simulink model "PhysicalEverSimmer"  (R2026a)
settings: Solver=VariableStepAuto  StopTime=14400
undefined symbols (not defined in the file): ES_PackRate_bph, ES_PrepRate_bph, ES_QCRate_bph, ES_Resupply_bph, Fault_T_Cell1, Fault_T_Cell2, Fault_T_Cell3, Recipe_Block_s, Recipe_Count, Resupply_Cutoff_T, Transport_Latency_s, Transport_Rate_bph
(part 2 of 2)

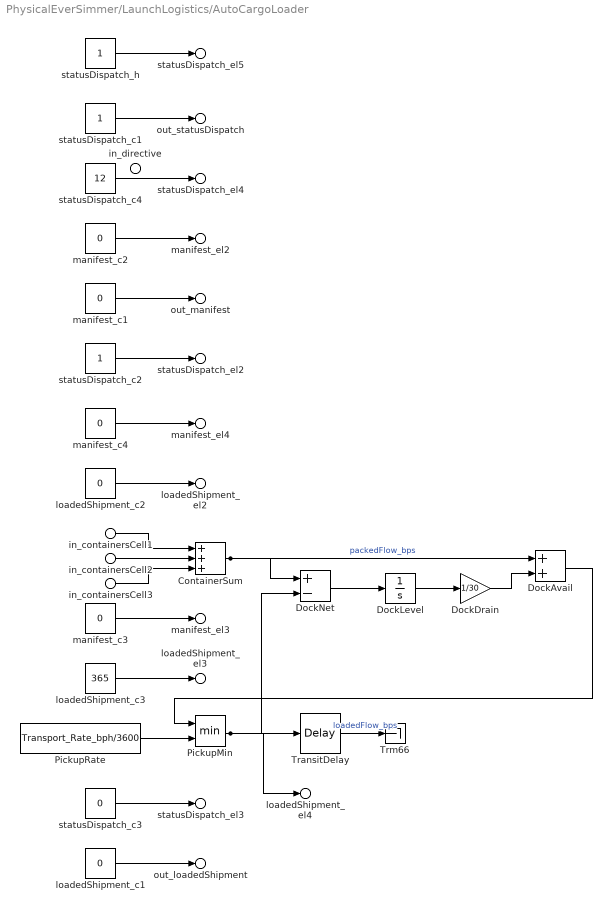
== system PhysicalEverSimmer/LaunchLogistics/AutoCargoLoader ==
  in_containersCell1 : Inport  PortName=containersCell1  Element=flow_bps
  in_containersCell2 : Inport  Port=2  PortName=containersCell2  Element=flow_bps
  in_containersCell3 : Inport  Port=3  PortName=containersCell3  Element=flow_bps
  in_directive : Inport  Port=4  PortName=directive
  ContainerSum : Sum  Inputs=+++
  DockAvail : Sum
  DockDrain : Gain  Gain=1/30
  DockLevel : Integrator  LimitOutput=on  UpperSaturationLimit=600  LowerSaturationLimit=0
  DockNet : Sum  Inputs=+-
  PickupMin : MinMax  Inputs=2
  PickupRate : Constant  Value=Transport_Rate_bph/3600
  TransitDelay : TransportDelay  DelayTime=Transport_Latency_s
  Trm66 : Terminator
  loadedShipment_c1 : Constant  Value=0
  loadedShipment_c2 : Constant  Value=0
  loadedShipment_c3 : Constant  Value=365
  manifest_c{1..4} (4 alike) : Constant  Value=0
  statusDispatch_c1 : Constant
  statusDispatch_c2 : Constant
  statusDispatch_c3 : Constant  Value=0
  statusDispatch_c4 : Constant  Value=12
  statusDispatch_h : Constant
  out_loadedShipment : Outport  PortName=loadedShipment  Element=batchId
  loadedShipment_el2 : Outport  PortName=loadedShipment  Element=count
  loadedShipment_el3 : Outport  PortName=loadedShipment  Element=sealRating_days
  loadedShipment_el4 : Outport  PortName=loadedShipment  Element=flow_bps
  out_manifest : Outport  Port=2  PortName=manifest  Element=destinationId
  manifest_el2 : Outport  Port=2  PortName=manifest  Element=batchId
  manifest_el3 : Outport  Port=2  PortName=manifest  Element=count
  manifest_el4 : Outport  Port=2  PortName=manifest  Element=mass_kg
  out_statusDispatch : Outport  Port=3  PortName=statusDispatch  Element=unitId
  statusDispatch_el2 : Outport  Port=3  PortName=statusDispatch  Element=opState
  statusDispatch_el3 : Outport  Port=3  PortName=statusDispatch  Element=faultCode
  statusDispatch_el4 : Outport  Port=3  PortName=statusDispatch  Element=power_kW
  statusDispatch_el5 : Outport  Port=3  PortName=statusDispatch  Element=health
  wires:
  manifest_c1/1 -> out_manifest/1
  statusDispatch_h/1 -> statusDispatch_el5/1
  statusDispatch_c1/1 -> out_statusDispatch/1
  statusDispatch_c4/1 -> statusDispatch_el4/1
  loadedShipment_c2/1 -> loadedShipment_el2/1
  manifest_c2/1 -> manifest_el2/1
  statusDispatch_c2/1 -> statusDispatch_el2/1
  manifest_c4/1 -> manifest_el4/1
  in_containersCell1/1 -> ContainerSum/1
  manifest_c3/1 -> manifest_el3/1
  in_containersCell2/1 -> ContainerSum/2
  in_containersCell3/1 -> ContainerSum/3
  loadedShipment_c3/1 -> loadedShipment_el3/1
  PickupRate/1 -> PickupMin/2
  loadedShipment_c1/1 -> out_loadedShipment/1
  statusDispatch_c3/1 -> statusDispatch_el3/1
  ContainerSum/1 -> DockAvail/1, DockNet/1  "packedFlow_bps"
  PickupMin/1 -> DockNet/2, TransitDelay/1, loadedShipment_el4/1
  DockNet/1 -> DockLevel/1
  TransitDelay/1 -> Trm66/1  "loadedFlow_bps"
  DockLevel/1 -> DockDrain/1
  DockDrain/1 -> DockAvail/2
  DockAvail/1 -> PickupMin/1

== system PhysicalEverSimmer/LaunchLogistics/AutoRefuelCell ==
  in_directive : Inport  PortName=directive
  statusRefuel_c1 : Constant
  statusRefuel_c2 : Constant
  statusRefuel_c3 : Constant  Value=0
  statusRefuel_c4 : Constant  Value=10
  statusRefuel_h : Constant
  out_statusRefuel : Outport  PortName=statusRefuel  Element=unitId
  statusRefuel_el2 : Outport  PortName=statusRefuel  Element=opState
  statusRefuel_el3 : Outport  PortName=statusRefuel  Element=faultCode
  statusRefuel_el4 : Outport  PortName=statusRefuel  Element=power_kW
  statusRefuel_el5 : Outport  PortName=statusRefuel  Element=health
  wires:
  statusRefuel_h/1 -> statusRefuel_el5/1
  statusRefuel_c3/1 -> statusRefuel_el3/1
  statusRefuel_c1/1 -> out_statusRefuel/1
  statusRefuel_c4/1 -> statusRefuel_el4/1
  statusRefuel_c2/1 -> statusRefuel_el2/1

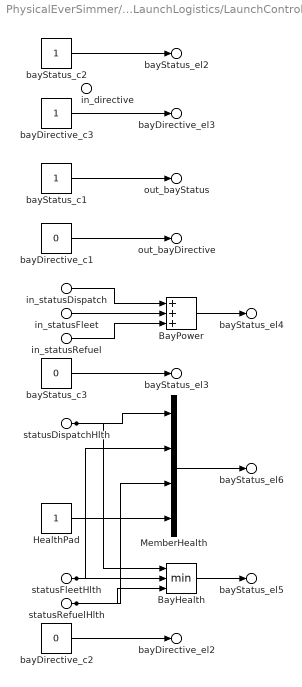
== system PhysicalEverSimmer/LaunchLogistics/LaunchController ==
  in_directive : Inport  PortName=directive
  in_statusDispatch : Inport  Port=2  PortName=statusDispatch  Element=power_kW
  statusDispatchHlth : Inport  Port=2  PortName=statusDispatch  Element=health
  in_statusRefuel : Inport  Port=3  PortName=statusRefuel  Element=power_kW
  statusRefuelHlth : Inport  Port=3  PortName=statusRefuel  Element=health
  in_statusFleet : Inport  Port=4  PortName=statusFleet  Element=power_kW
  statusFleetHlth : Inport  Port=4  PortName=statusFleet  Element=health
  BayHealth : MinMax  Inputs=3
  BayPower : Sum  Inputs=+++
  HealthPad : Constant
  MemberHealth : Mux
  bayDirective_c1 : Constant  Value=0
  bayDirective_c2 : Constant  Value=0
  bayDirective_c3 : Constant
  bayStatus_c1 : Constant
  bayStatus_c2 : Constant
  bayStatus_c3 : Constant  Value=0
  out_bayDirective : Outport  PortName=bayDirective  Element=cmdType
  bayDirective_el2 : Outport  PortName=bayDirective  Element=targetId
  bayDirective_el3 : Outport  PortName=bayDirective  Element=setpoint
  out_bayStatus : Outport  Port=2  PortName=bayStatus  Element=unitId
  bayStatus_el2 : Outport  Port=2  PortName=bayStatus  Element=opState
  bayStatus_el3 : Outport  Port=2  PortName=bayStatus  Element=faultCode
  bayStatus_el4 : Outport  Port=2  PortName=bayStatus  Element=power_kW
  bayStatus_el5 : Outport  Port=2  PortName=bayStatus  Element=health
  bayStatus_el6 : Outport  Port=2  PortName=bayStatus  Element=lineHealth
  wires:
  bayDirective_c1/1 -> out_bayDirective/1
  bayStatus_c2/1 -> bayStatus_el2/1
  bayDirective_c3/1 -> bayDirective_el3/1
  bayStatus_c1/1 -> out_bayStatus/1
  in_statusFleet/1 -> BayPower/2
  in_statusDispatch/1 -> BayPower/1
  bayStatus_c3/1 -> bayStatus_el3/1
  bayDirective_c2/1 -> bayDirective_el2/1
  in_statusRefuel/1 -> BayPower/3
  statusDispatchHlth/1 -> BayHealth/1, MemberHealth/1
  HealthPad/1 -> MemberHealth/4
  statusFleetHlth/1 -> BayHealth/2, MemberHealth/2
  statusRefuelHlth/1 -> BayHealth/3, MemberHealth/3
  BayPower/1 -> bayStatus_el4/1
  MemberHealth/1 -> bayStatus_el6/1
  BayHealth/1 -> bayStatus_el5/1

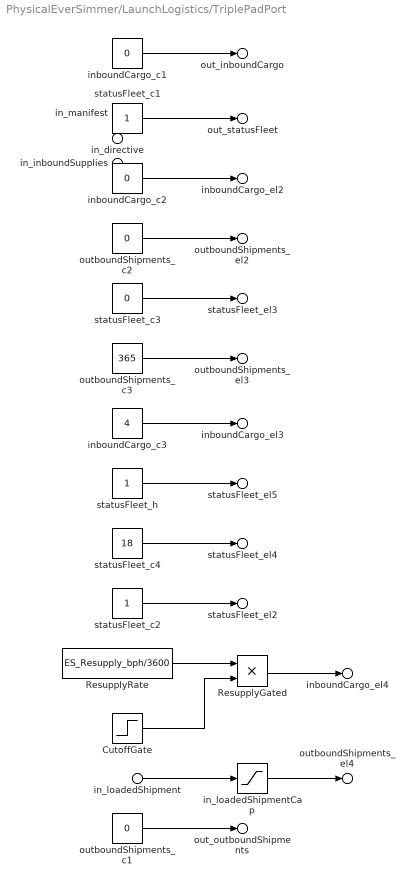
== system PhysicalEverSimmer/LaunchLogistics/TriplePadPort ==
  in_loadedShipment : Inport  PortName=loadedShipment  Element=flow_bps
  in_manifest : Inport  Port=2  PortName=manifest
  in_directive : Inport  Port=3  PortName=directive
  in_inboundSupplies : Inport  Port=4  PortName=inboundSupplies
  CutoffGate : Step  Time=Resupply_Cutoff_T  InitialValue=1  FinalValue=0  SampleTime=0
  ResupplyGated : Product
  ResupplyRate : Constant  Value=ES_Resupply_bph/3600
  in_loadedShipmentCap : Saturate  UpperLimit=0.0777777777778  LowerLimit=0
  inboundCargo_c1 : Constant  Value=0
  inboundCargo_c2 : Constant  Value=0
  inboundCargo_c3 : Constant  Value=4
  outboundShipments_c1 : Constant  Value=0
  outboundShipments_c2 : Constant  Value=0
  outboundShipments_c3 : Constant  Value=365
  statusFleet_c1 : Constant
  statusFleet_c2 : Constant
  statusFleet_c3 : Constant  Value=0
  statusFleet_c4 : Constant  Value=18
  statusFleet_h : Constant
  out_inboundCargo : Outport  PortName=inboundCargo  Element=palletId
  inboundCargo_el2 : Outport  PortName=inboundCargo  Element=mass_kg
  inboundCargo_el3 : Outport  PortName=inboundCargo  Element=temp_C
  inboundCargo_el4 : Outport  PortName=inboundCargo  Element=flow_bps
  out_outboundShipments : Outport  Port=2  PortName=outboundShipments  Element=batchId
  outboundShipments_el2 : Outport  Port=2  PortName=outboundShipments  Element=count
  outboundShipments_el3 : Outport  Port=2  PortName=outboundShipments  Element=sealRating_days
  outboundShipments_el4 : Outport  Port=2  PortName=outboundShipments  Element=flow_bps
  out_statusFleet : Outport  Port=3  PortName=statusFleet  Element=unitId
  statusFleet_el2 : Outport  Port=3  PortName=statusFleet  Element=opState
  statusFleet_el3 : Outport  Port=3  PortName=statusFleet  Element=faultCode
  statusFleet_el4 : Outport  Port=3  PortName=statusFleet  Element=power_kW
  statusFleet_el5 : Outport  Port=3  PortName=statusFleet  Element=health
  wires:
  inboundCargo_c1/1 -> out_inboundCargo/1
  statusFleet_c1/1 -> out_statusFleet/1
  statusFleet_h/1 -> statusFleet_el5/1
  inboundCargo_c2/1 -> inboundCargo_el2/1
  inboundCargo_c3/1 -> inboundCargo_el3/1
  outboundShipments_c2/1 -> outboundShipments_el2/1
  outboundShipments_c3/1 -> outboundShipments_el3/1
  statusFleet_c3/1 -> statusFleet_el3/1
  statusFleet_c4/1 -> statusFleet_el4/1
  statusFleet_c2/1 -> statusFleet_el2/1
  ResupplyRate/1 -> ResupplyGated/1
  CutoffGate/1 -> ResupplyGated/2
  in_loadedShipment/1 -> in_loadedShipmentCap/1
  outboundShipments_c1/1 -> out_outboundShipments/1
  ResupplyGated/1 -> inboundCargo_el4/1
  in_loadedShipmentCap/1 -> outboundShipments_el4/1

== system PhysicalEverSimmer/PlantServices/GravityCompMesh ==
  in_ambientGravity : Inport  PortName=ambientGravity  Element=gravity_g
  envStatus_c1 : Constant  Value=100
  out_envStatus : Outport  PortName=envStatus  Element=gravity_g
  envStatus_el2 : Outport  PortName=envStatus  Element=compensation_pct
  wires:
  in_ambientGravity/1 -> out_envStatus/1  "ambientGravity"
  envStatus_c1/1 -> envStatus_el2/1

== system PhysicalEverSimmer/PlantServices/RedundantReactorPair ==
  in_directive : Inport  PortName=directive
  statusPower_c1 : Constant
  statusPower_c2 : Constant
  statusPower_c3 : Constant  Value=0
  statusPower_c4 : Constant  Value=0
  statusPower_h : Constant
  out_statusPower : Outport  PortName=statusPower  Element=unitId
  statusPower_el2 : Outport  PortName=statusPower  Element=opState
  statusPower_el3 : Outport  PortName=statusPower  Element=faultCode
  statusPower_el4 : Outport  PortName=statusPower  Element=power_kW
  statusPower_el5 : Outport  PortName=statusPower  Element=health
  wires:
  statusPower_h/1 -> statusPower_el5/1
  statusPower_c3/1 -> statusPower_el3/1
  statusPower_c1/1 -> out_statusPower/1
  statusPower_c4/1 -> statusPower_el4/1
  statusPower_c2/1 -> statusPower_el2/1

== system PhysicalEverSimmer/PlantServices/RoboTransportSwarm ==
  in_transportDirective : Inport  PortName=transportDirective
  statusTransport_c1 : Constant
  statusTransport_c2 : Constant
  statusTransport_c3 : Constant  Value=0
  statusTransport_c4 : Constant  Value=15
  statusTransport_h : Constant
  out_statusTransport : Outport  PortName=statusTransport  Element=unitId
  statusTransport_el2 : Outport  PortName=statusTransport  Element=opState
  statusTransport_el3 : Outport  PortName=statusTransport  Element=faultCode
  statusTransport_el4 : Outport  PortName=statusTransport  Element=power_kW
  statusTransport_el5 : Outport  PortName=statusTransport  Element=health
  wires:
  statusTransport_h/1 -> statusTransport_el5/1
  statusTransport_c3/1 -> statusTransport_el3/1
  statusTransport_c1/1 -> out_statusTransport/1
  statusTransport_c4/1 -> statusTransport_el4/1
  statusTransport_c2/1 -> statusTransport_el2/1

== system PhysicalEverSimmer/PlantServices/ServicesController ==
  in_directive : Inport  PortName=directive
  in_statusPower : Inport  Port=2  PortName=statusPower  Element=power_kW
  statusPowerHlth : Inport  Port=2  PortName=statusPower  Element=health
  in_statusTransport : Inport  Port=3  PortName=statusTransport  Element=power_kW
  statusTransportHlth : Inport  Port=3  PortName=statusTransport  Element=health
  BayHealth : MinMax  Inputs=2
  BayPower : Sum
  HealthPad : Constant
  MemberHealth : Mux
  bayDirective_c1 : Constant  Value=0
  bayDirective_c2 : Constant  Value=0
  bayDirective_c3 : Constant
  bayStatus_c1 : Constant
  bayStatus_c2 : Constant
  bayStatus_c3 : Constant  Value=0
  out_bayDirective : Outport  PortName=bayDirective  Element=cmdType
  bayDirective_el2 : Outport  PortName=bayDirective  Element=targetId
  bayDirective_el3 : Outport  PortName=bayDirective  Element=setpoint
  out_bayStatus : Outport  Port=2  PortName=bayStatus  Element=unitId
  bayStatus_el2 : Outport  Port=2  PortName=bayStatus  Element=opState
  bayStatus_el3 : Outport  Port=2  PortName=bayStatus  Element=faultCode
  bayStatus_el4 : Outport  Port=2  PortName=bayStatus  Element=power_kW
  bayStatus_el5 : Outport  Port=2  PortName=bayStatus  Element=health
  bayStatus_el6 : Outport  Port=2  PortName=bayStatus  Element=lineHealth
  wires:
  bayStatus_c2/1 -> bayStatus_el2/1
  bayDirective_c3/1 -> bayDirective_el3/1
  statusPowerHlth/1 -> BayHealth/1, MemberHealth/1
  bayStatus_c1/1 -> out_bayStatus/1
  bayDirective_c1/1 -> out_bayDirective/1
  bayStatus_c3/1 -> bayStatus_el3/1
  in_statusPower/1 -> BayPower/1
  in_statusTransport/1 -> BayPower/2
  HealthPad/1 -> MemberHealth/3, MemberHealth/4
  statusTransportHlth/1 -> BayHealth/2, MemberHealth/2
  bayDirective_c2/1 -> bayDirective_el2/1
  BayPower/1 -> bayStatus_el4/1
  MemberHealth/1 -> bayStatus_el6/1
  BayHealth/1 -> bayStatus_el5/1

== system PhysicalEverSimmer/ProductionCell1/CellController ==
  in_directive : Inport  PortName=directive
  statusPrepPwr : Inport  Port=2  PortName=statusPrep  Element=power_kW
  in_statusPrep : Inport  Port=2  PortName=statusPrep  Element=health
  statusCookPwr : Inport  Port=3  PortName=statusCook  Element=power_kW
  in_statusCook : Inport  Port=3  PortName=statusCook  Element=health
  statusQAPwr : Inport  Port=4  PortName=statusQA  Element=power_kW
  in_statusQA : Inport  Port=4  PortName=statusQA  Element=health
  statusPackPwr : Inport  Port=5  PortName=statusPack  Element=power_kW
  in_statusPack : Inport  Port=5  PortName=statusPack  Element=health
  HealthMin : MinMax  Inputs=4
  OwnPower : Constant  Value=2
  PowerSum : Sum  Inputs=+++++
  cellDirective_c1 : Constant  Value=0
  cellDirective_c2 : Constant  Value=0
  cellDirective_c3 : Constant
  statusCell_c1 : Constant
  statusCell_c2 : Constant
  statusCell_c3 : Constant  Value=0
  out_cellDirective : Outport  PortName=cellDirective  Element=cmdType
  cellDirective_el2 : Outport  PortName=cellDirective  Element=targetId
  cellDirective_el3 : Outport  PortName=cellDirective  Element=setpoint
  out_statusCell : Outport  Port=2  PortName=statusCell  Element=unitId
  statusCell_el2 : Outport  Port=2  PortName=statusCell  Element=opState
  statusCell_el3 : Outport  Port=2  PortName=statusCell  Element=faultCode
  statusCell_el4 : Outport  Port=2  PortName=statusCell  Element=power_kW
  statusCell_el5 : Outport  Port=2  PortName=statusCell  Element=health
  wires:
  cellDirective_c1/1 -> out_cellDirective/1
  statusCookPwr/1 -> PowerSum/2
  cellDirective_c2/1 -> cellDirective_el2/1
  statusCell_c2/1 -> statusCell_el2/1
  statusQAPwr/1 -> PowerSum/3
  statusPrepPwr/1 -> PowerSum/1
  statusCell_c3/1 -> statusCell_el3/1
  cellDirective_c3/1 -> cellDirective_el3/1
  statusPackPwr/1 -> PowerSum/4
  OwnPower/1 -> PowerSum/5
  in_statusPrep/1 -> HealthMin/1
  in_statusCook/1 -> HealthMin/2
  in_statusQA/1 -> HealthMin/3
  PowerSum/1 -> statusCell_el4/1
  in_statusPack/1 -> HealthMin/4
  statusCell_c1/1 -> out_statusCell/1
  HealthMin/1 -> statusCell_el5/1

== system PhysicalEverSimmer/ProductionCell1/CellCookVat ==
  in_preppedBatch : Inport  PortName=preppedBatch  Element=flow_bps
  in_directive : Inport  Port=2  PortName=directive  Element=setpoint
  En_Gate_Fault_T_Cell1 : Product
  Gate_Fault_T_Cell1 : Step  Time=Fault_T_Cell1  InitialValue=1  FinalValue=0  SampleTime=0
  StateDbl : DataTypeConversion  OutDataTypeStr=double  SaturateOnIntegerOverflow=off  RndMeth=Floor
  ToLitres : Gain  Gain=1800
  Trm37 : Terminator
  Vat : ModelReference  ModelNameDialog=BehCookVat  UsingDefaultArgumentValue=0,0,0,0,0,0,0,0  SimulationMode=Normal  ModelReferenceVersion=1.15
  cookedSoup_c1 : Constant  Value=0
  cookedSoup_c2 : Constant  Value=0
  statusCook_c1 : Constant
  statusCook_c2 : Constant  Value=0
  out_cookedSoup : Outport  PortName=cookedSoup  Element=batchId
  cookedSoup_el2 : Outport  PortName=cookedSoup  Element=volume_L
  cookedSoup_el3 : Outport  PortName=cookedSoup  Element=temp_C
  cookedSoup_el4 : Outport  PortName=cookedSoup  Element=contamination_ppm
  cookedSoup_el5 : Outport  PortName=cookedSoup  Element=flow_bps
  out_statusCook : Outport  Port=2  PortName=statusCook  Element=unitId
  statusCook_el2 : Outport  Port=2  PortName=statusCook  Element=opState
  statusCook_el3 : Outport  Port=2  PortName=statusCook  Element=faultCode
  statusCook_el4 : Outport  Port=2  PortName=statusCook  Element=power_kW
  statusCook_el5 : Outport  Port=2  PortName=statusCook  Element=health
  wires:
  cookedSoup_c2/1 -> cookedSoup_el4/1
  in_preppedBatch/1 -> Vat/1
  Gate_Fault_T_Cell1/1 -> En_Gate_Fault_T_Cell1/2, statusCook_el5/1
  statusCook_c2/1 -> statusCook_el3/1
  En_Gate_Fault_T_Cell1/1 -> Vat/2
  statusCook_c1/1 -> out_statusCook/1
  in_directive/1 -> En_Gate_Fault_T_Cell1/1
  cookedSoup_c1/1 -> out_cookedSoup/1
  Vat/1 -> ToLitres/1, cookedSoup_el5/1  "soupFlow_Cell1"
  Vat/2 -> statusCook_el4/1
  Vat/3 -> cookedSoup_el3/1  "vatTemp_Cell1"
  Vat/4 -> StateDbl/1  "vatState_Cell1"
  Vat/5 -> Trm37/1
  ToLitres/1 -> cookedSoup_el2/1
  StateDbl/1 -> statusCook_el2/1

== system PhysicalEverSimmer/ProductionCell1/CellPackager ==
  in_approvedSoup : Inport  PortName=approvedSoup  Element=flow_bps
  in_directive : Inport  Port=2  PortName=directive  Element=setpoint
  En_Gate_Fault_T_Cell1 : Product
  Gate_Fault_T_Cell1 : Step  Time=Fault_T_Cell1  InitialValue=1  FinalValue=0  SampleTime=0
  Pack : ModelReference  ModelNameDialog=BehPackager  UsingDefaultArgumentValue=0,0  SimulationMode=Normal  ModelReferenceVersion=1.5
  PackDraw : Constant  Value=ES_PackRate_bph/3600
  Surge : ModelReference  ModelNameDialog=BehStorage  UsingDefaultArgumentValue=0,0  SimulationMode=Normal  ModelReferenceVersion=1.4
  Trm44 : Terminator
  Trm45 : Terminator
  sealedContainers_c1 : Constant  Value=0
  sealedContainers_c2 : Constant  Value=0
  sealedContainers_c3 : Constant  Value=365
  statusPack_c1 : Constant
  statusPack_c2 : Constant
  statusPack_c3 : Constant  Value=0
  statusPack_c4 : Constant  Value=12
  out_sealedContainers : Outport  PortName=sealedContainers  Element=batchId
  sealedContainers_el2 : Outport  PortName=sealedContainers  Element=count
  sealedContainers_el3 : Outport  PortName=sealedContainers  Element=sealRating_days
  sealedContainers_el4 : Outport  PortName=sealedContainers  Element=flow_bps
  out_statusPack : Outport  Port=2  PortName=statusPack  Element=unitId
  statusPack_el2 : Outport  Port=2  PortName=statusPack  Element=opState
  statusPack_el3 : Outport  Port=2  PortName=statusPack  Element=faultCode
  statusPack_el4 : Outport  Port=2  PortName=statusPack  Element=power_kW
  statusPack_el5 : Outport  Port=2  PortName=statusPack  Element=health
  wires:
  statusPack_c2/1 -> statusPack_el2/1
  in_directive/1 -> En_Gate_Fault_T_Cell1/1
  sealedContainers_c1/1 -> out_sealedContainers/1
  sealedContainers_c3/1 -> sealedContainers_el3/1
  statusPack_c4/1 -> statusPack_el4/1
  statusPack_c1/1 -> out_statusPack/1
  Gate_Fault_T_Cell1/1 -> En_Gate_Fault_T_Cell1/2, statusPack_el5/1
  statusPack_c3/1 -> statusPack_el3/1
  in_approvedSoup/1 -> Surge/1
  PackDraw/1 -> Surge/2
  sealedContainers_c2/1 -> sealedContainers_el2/1
  En_Gate_Fault_T_Cell1/1 -> Pack/2
  Surge/1 -> Pack/1
  Surge/2 -> Trm44/1
  Surge/3 -> Trm45/1
  Pack/1 -> sealedContainers_el4/1

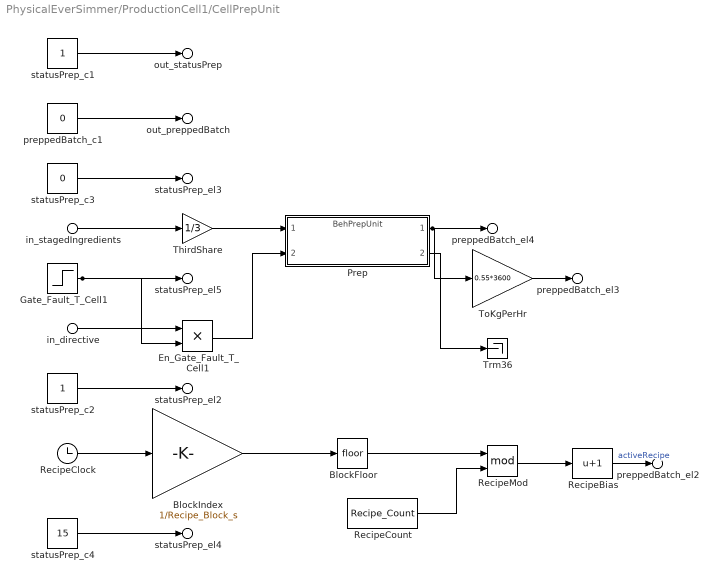
== system PhysicalEverSimmer/ProductionCell1/CellPrepUnit ==
  in_stagedIngredients : Inport  PortName=stagedIngredients  Element=flow_bps
  in_directive : Inport  Port=2  PortName=directive  Element=setpoint
  BlockFloor : Rounding
  BlockIndex : Gain  Gain=1/Recipe_Block_s
  En_Gate_Fault_T_Cell1 : Product
  Gate_Fault_T_Cell1 : Step  Time=Fault_T_Cell1  InitialValue=1  FinalValue=0  SampleTime=0
  Prep : ModelReference  ModelNameDialog=BehPrepUnit  UsingDefaultArgumentValue=0,0  SimulationMode=Normal  ModelReferenceVersion=1.5
  RecipeBias : Bias  Bias=1  SaturateOnIntegerOverflow=off
  RecipeClock : Clock
  RecipeCount : Constant  Value=Recipe_Count
  RecipeMod : Math  Operator=mod
  ThirdShare : Gain  Gain=1/3
  ToKgPerHr : Gain  Gain=0.55*3600
  Trm36 : Terminator
  preppedBatch_c1 : Constant  Value=0
  statusPrep_c1 : Constant
  statusPrep_c2 : Constant
  statusPrep_c3 : Constant  Value=0
  statusPrep_c4 : Constant  Value=15
  out_preppedBatch : Outport  PortName=preppedBatch  Element=batchId
  preppedBatch_el2 : Outport  PortName=preppedBatch  Element=recipeId
  preppedBatch_el3 : Outport  PortName=preppedBatch  Element=mass_kg
  preppedBatch_el4 : Outport  PortName=preppedBatch  Element=flow_bps
  out_statusPrep : Outport  Port=2  PortName=statusPrep  Element=unitId
  statusPrep_el2 : Outport  Port=2  PortName=statusPrep  Element=opState
  statusPrep_el3 : Outport  Port=2  PortName=statusPrep  Element=faultCode
  statusPrep_el4 : Outport  Port=2  PortName=statusPrep  Element=power_kW
  statusPrep_el5 : Outport  Port=2  PortName=statusPrep  Element=health
  wires:
  in_directive/1 -> En_Gate_Fault_T_Cell1/1
  Prep/1 -> preppedBatch_el4/1, ToKgPerHr/1
  statusPrep_c1/1 -> out_statusPrep/1
  preppedBatch_c1/1 -> out_preppedBatch/1
  RecipeMod/1 -> RecipeBias/1
  statusPrep_c3/1 -> statusPrep_el3/1
  statusPrep_c2/1 -> statusPrep_el2/1
  in_stagedIngredients/1 -> ThirdShare/1
  Gate_Fault_T_Cell1/1 -> En_Gate_Fault_T_Cell1/2, statusPrep_el5/1
  RecipeClock/1 -> BlockIndex/1
  statusPrep_c4/1 -> statusPrep_el4/1
  ThirdShare/1 -> Prep/1
  En_Gate_Fault_T_Cell1/1 -> Prep/2
  BlockIndex/1 -> BlockFloor/1
  Prep/2 -> Trm36/1
  BlockFloor/1 -> RecipeMod/1
  RecipeCount/1 -> RecipeMod/2
  ToKgPerHr/1 -> preppedBatch_el3/1
  RecipeBias/1 -> preppedBatch_el2/1  "activeRecipe"

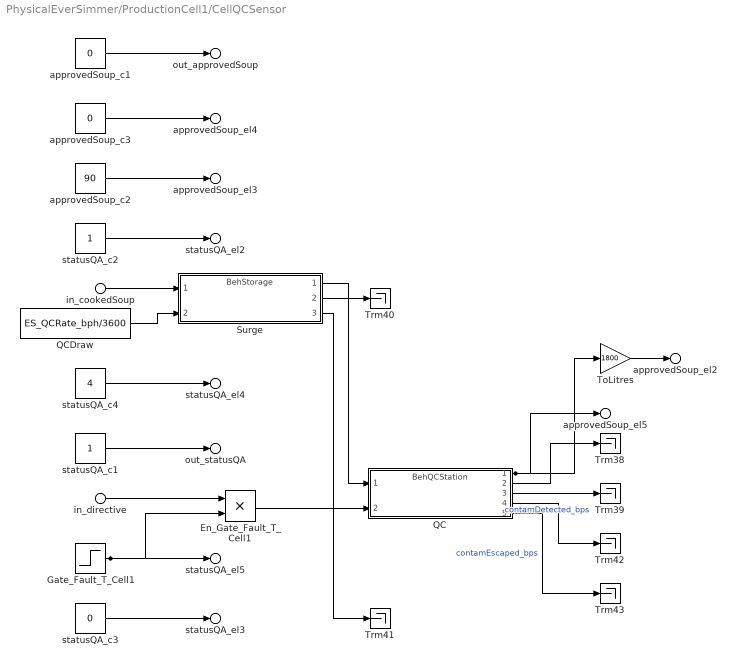
== system PhysicalEverSimmer/ProductionCell1/CellQCSensor ==
  in_cookedSoup : Inport  PortName=cookedSoup  Element=flow_bps
  in_directive : Inport  Port=2  PortName=directive  Element=setpoint
  En_Gate_Fault_T_Cell1 : Product
  Gate_Fault_T_Cell1 : Step  Time=Fault_T_Cell1  InitialValue=1  FinalValue=0  SampleTime=0
  QC : ModelReference  ModelNameDialog=BehQCStation  UsingDefaultArgumentValue=0,0,0,0,0,0  SimulationMode=Normal  ModelReferenceVersion=1.6
  QCDraw : Constant  Value=ES_QCRate_bph/3600
  Surge : ModelReference  ModelNameDialog=BehStorage  UsingDefaultArgumentValue=0,0  SimulationMode=Normal  ModelReferenceVersion=1.4
  ToLitres : Gain  Gain=1800
  Trm{38..43} (6 alike) : Terminator
  approvedSoup_c1 : Constant  Value=0
  approvedSoup_c2 : Constant  Value=90
  approvedSoup_c3 : Constant  Value=0
  statusQA_c1 : Constant
  statusQA_c2 : Constant
  statusQA_c3 : Constant  Value=0
  statusQA_c4 : Constant  Value=4
  out_approvedSoup : Outport  PortName=approvedSoup  Element=batchId
  approvedSoup_el2 : Outport  PortName=approvedSoup  Element=volume_L
  approvedSoup_el3 : Outport  PortName=approvedSoup  Element=temp_C
  approvedSoup_el4 : Outport  PortName=approvedSoup  Element=contamination_ppm
  approvedSoup_el5 : Outport  PortName=approvedSoup  Element=flow_bps
  out_statusQA : Outport  Port=2  PortName=statusQA  Element=unitId
  statusQA_el2 : Outport  Port=2  PortName=statusQA  Element=opState
  statusQA_el3 : Outport  Port=2  PortName=statusQA  Element=faultCode
  statusQA_el4 : Outport  Port=2  PortName=statusQA  Element=power_kW
  statusQA_el5 : Outport  Port=2  PortName=statusQA  Element=health
  wires:
  in_cookedSoup/1 -> Surge/1
  approvedSoup_c1/1 -> out_approvedSoup/1
  approvedSoup_c3/1 -> approvedSoup_el4/1
  QCDraw/1 -> Surge/2
  approvedSoup_c2/1 -> approvedSoup_el3/1
  statusQA_c2/1 -> statusQA_el2/1
  statusQA_c1/1 -> out_statusQA/1
  statusQA_c4/1 -> statusQA_el4/1
  En_Gate_Fault_T_Cell1/1 -> QC/2
  in_directive/1 -> En_Gate_Fault_T_Cell1/1
  Gate_Fault_T_Cell1/1 -> En_Gate_Fault_T_Cell1/2, statusQA_el5/1
  statusQA_c3/1 -> statusQA_el3/1
  Surge/1 -> QC/1
  Surge/2 -> Trm40/1
  Surge/3 -> Trm41/1
  QC/1 -> ToLitres/1, approvedSoup_el5/1
  QC/2 -> Trm38/1
  QC/3 -> Trm39/1
  ToLitres/1 -> approvedSoup_el2/1
  QC/4 -> Trm42/1  "contamDetected_bps"
  QC/5 -> Trm43/1  "contamEscaped_bps"

== system PhysicalEverSimmer/ProductionCell2/CellController ==
  in_directive : Inport  PortName=directive
  statusPrepPwr : Inport  Port=2  PortName=statusPrep  Element=power_kW
  in_statusPrep : Inport  Port=2  PortName=statusPrep  Element=health
  statusCookPwr : Inport  Port=3  PortName=statusCook  Element=power_kW
  in_statusCook : Inport  Port=3  PortName=statusCook  Element=health
  statusQAPwr : Inport  Port=4  PortName=statusQA  Element=power_kW
  in_statusQA : Inport  Port=4  PortName=statusQA  Element=health
  statusPackPwr : Inport  Port=5  PortName=statusPack  Element=power_kW
  in_statusPack : Inport  Port=5  PortName=statusPack  Element=health
  HealthMin : MinMax  Inputs=4
  OwnPower : Constant  Value=2
  PowerSum : Sum  Inputs=+++++
  cellDirective_c1 : Constant  Value=0
  cellDirective_c2 : Constant  Value=0
  cellDirective_c3 : Constant
  statusCell_c1 : Constant  Value=2
  statusCell_c2 : Constant
  statusCell_c3 : Constant  Value=0
  out_cellDirective : Outport  PortName=cellDirective  Element=cmdType
  cellDirective_el2 : Outport  PortName=cellDirective  Element=targetId
  cellDirective_el3 : Outport  PortName=cellDirective  Element=setpoint
  out_statusCell : Outport  Port=2  PortName=statusCell  Element=unitId
  statusCell_el2 : Outport  Port=2  PortName=statusCell  Element=opState
  statusCell_el3 : Outport  Port=2  PortName=statusCell  Element=faultCode
  statusCell_el4 : Outport  Port=2  PortName=statusCell  Element=power_kW
  statusCell_el5 : Outport  Port=2  PortName=statusCell  Element=health
  wires:
  statusQAPwr/1 -> PowerSum/3
  statusPrepPwr/1 -> PowerSum/1
  cellDirective_c1/1 -> out_cellDirective/1
  OwnPower/1 -> PowerSum/5
  cellDirective_c2/1 -> cellDirective_el2/1
  statusCookPwr/1 -> PowerSum/2
  statusCell_c2/1 -> statusCell_el2/1
  cellDirective_c3/1 -> cellDirective_el3/1
  statusCell_c3/1 -> statusCell_el3/1
  statusPackPwr/1 -> PowerSum/4
  in_statusPrep/1 -> HealthMin/1
  in_statusCook/1 -> HealthMin/2
  in_statusQA/1 -> HealthMin/3
  in_statusPack/1 -> HealthMin/4
  statusCell_c1/1 -> out_statusCell/1
  PowerSum/1 -> statusCell_el4/1
  HealthMin/1 -> statusCell_el5/1

== system PhysicalEverSimmer/ProductionCell2/CellCookVat ==
  in_preppedBatch : Inport  PortName=preppedBatch  Element=flow_bps
  in_directive : Inport  Port=2  PortName=directive  Element=setpoint
  En_Gate_Fault_T_Cell2 : Product
  Gate_Fault_T_Cell2 : Step  Time=Fault_T_Cell2  InitialValue=1  FinalValue=0  SampleTime=0
  StateDbl : DataTypeConversion  OutDataTypeStr=double  SaturateOnIntegerOverflow=off  RndMeth=Floor
  ToLitres : Gain  Gain=1800
  Trm47 : Terminator
  Vat : ModelReference  ModelNameDialog=BehCookVat  UsingDefaultArgumentValue=0,0,0,0,0,0,0,0  SimulationMode=Normal  ModelReferenceVersion=1.15
  cookedSoup_c1 : Constant  Value=0
  cookedSoup_c2 : Constant  Value=0
  statusCook_c1 : Constant  Value=2
  statusCook_c2 : Constant  Value=0
  out_cookedSoup : Outport  PortName=cookedSoup  Element=batchId
  cookedSoup_el2 : Outport  PortName=cookedSoup  Element=volume_L
  cookedSoup_el3 : Outport  PortName=cookedSoup  Element=temp_C
  cookedSoup_el4 : Outport  PortName=cookedSoup  Element=contamination_ppm
  cookedSoup_el5 : Outport  PortName=cookedSoup  Element=flow_bps
  out_statusCook : Outport  Port=2  PortName=statusCook  Element=unitId
  statusCook_el2 : Outport  Port=2  PortName=statusCook  Element=opState
  statusCook_el3 : Outport  Port=2  PortName=statusCook  Element=faultCode
  statusCook_el4 : Outport  Port=2  PortName=statusCook  Element=power_kW
  statusCook_el5 : Outport  Port=2  PortName=statusCook  Element=health
  wires:
  cookedSoup_c2/1 -> cookedSoup_el4/1
  Vat/5 -> Trm47/1
  in_directive/1 -> En_Gate_Fault_T_Cell2/1
  statusCook_c2/1 -> statusCook_el3/1
  En_Gate_Fault_T_Cell2/1 -> Vat/2
  Vat/3 -> cookedSoup_el3/1
  in_preppedBatch/1 -> Vat/1
  ToLitres/1 -> cookedSoup_el2/1
  statusCook_c1/1 -> out_statusCook/1
  cookedSoup_c1/1 -> out_cookedSoup/1
  Gate_Fault_T_Cell2/1 -> En_Gate_Fault_T_Cell2/2, statusCook_el5/1
  Vat/1 -> cookedSoup_el5/1, ToLitres/1  "soupFlow_Cell2"
  Vat/2 -> statusCook_el4/1
  Vat/4 -> StateDbl/1
  StateDbl/1 -> statusCook_el2/1

== system PhysicalEverSimmer/ProductionCell2/CellPackager ==
  in_approvedSoup : Inport  PortName=approvedSoup  Element=flow_bps
  in_directive : Inport  Port=2  PortName=directive  Element=setpoint
  En_Gate_Fault_T_Cell2 : Product
  Gate_Fault_T_Cell2 : Step  Time=Fault_T_Cell2  InitialValue=1  FinalValue=0  SampleTime=0
  Pack : ModelReference  ModelNameDialog=BehPackager  UsingDefaultArgumentValue=0,0  SimulationMode=Normal  ModelReferenceVersion=1.5
  PackDraw : Constant  Value=ES_PackRate_bph/3600
  Surge : ModelReference  ModelNameDialog=BehStorage  UsingDefaultArgumentValue=0,0  SimulationMode=Normal  ModelReferenceVersion=1.4
  Trm54 : Terminator
  Trm55 : Terminator
  sealedContainers_c1 : Constant  Value=0
  sealedContainers_c2 : Constant  Value=0
  sealedContainers_c3 : Constant  Value=365
  statusPack_c1 : Constant
  statusPack_c2 : Constant
  statusPack_c3 : Constant  Value=0
  statusPack_c4 : Constant  Value=12
  out_sealedContainers : Outport  PortName=sealedContainers  Element=batchId
  sealedContainers_el2 : Outport  PortName=sealedContainers  Element=count
  sealedContainers_el3 : Outport  PortName=sealedContainers  Element=sealRating_days
  sealedContainers_el4 : Outport  PortName=sealedContainers  Element=flow_bps
  out_statusPack : Outport  Port=2  PortName=statusPack  Element=unitId
  statusPack_el2 : Outport  Port=2  PortName=statusPack  Element=opState
  statusPack_el3 : Outport  Port=2  PortName=statusPack  Element=faultCode
  statusPack_el4 : Outport  Port=2  PortName=statusPack  Element=power_kW
  statusPack_el5 : Outport  Port=2  PortName=statusPack  Element=health
  wires:
  in_directive/1 -> En_Gate_Fault_T_Cell2/1
  statusPack_c2/1 -> statusPack_el2/1
  sealedContainers_c1/1 -> out_sealedContainers/1
  sealedContainers_c3/1 -> sealedContainers_el3/1
  statusPack_c1/1 -> out_statusPack/1
  statusPack_c4/1 -> statusPack_el4/1
  statusPack_c3/1 -> statusPack_el3/1
  Gate_Fault_T_Cell2/1 -> En_Gate_Fault_T_Cell2/2, statusPack_el5/1
  in_approvedSoup/1 -> Surge/1
  PackDraw/1 -> Surge/2
  sealedContainers_c2/1 -> sealedContainers_el2/1
  En_Gate_Fault_T_Cell2/1 -> Pack/2
  Surge/1 -> Pack/1
  Surge/2 -> Trm54/1
  Surge/3 -> Trm55/1
  Pack/1 -> sealedContainers_el4/1

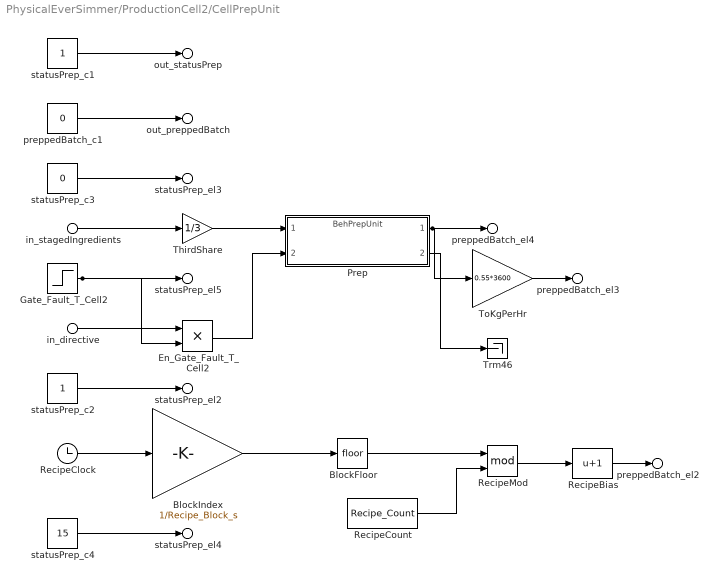
== system PhysicalEverSimmer/ProductionCell2/CellPrepUnit ==
  in_stagedIngredients : Inport  PortName=stagedIngredients  Element=flow_bps
  in_directive : Inport  Port=2  PortName=directive  Element=setpoint
  BlockFloor : Rounding
  BlockIndex : Gain  Gain=1/Recipe_Block_s
  En_Gate_Fault_T_Cell2 : Product
  Gate_Fault_T_Cell2 : Step  Time=Fault_T_Cell2  InitialValue=1  FinalValue=0  SampleTime=0
  Prep : ModelReference  ModelNameDialog=BehPrepUnit  UsingDefaultArgumentValue=0,0  SimulationMode=Normal  ModelReferenceVersion=1.5
  RecipeBias : Bias  Bias=1  SaturateOnIntegerOverflow=off
  RecipeClock : Clock
  RecipeCount : Constant  Value=Recipe_Count
  RecipeMod : Math  Operator=mod
  ThirdShare : Gain  Gain=1/3
  ToKgPerHr : Gain  Gain=0.55*3600
  Trm46 : Terminator
  preppedBatch_c1 : Constant  Value=0
  statusPrep_c1 : Constant
  statusPrep_c2 : Constant
  statusPrep_c3 : Constant  Value=0
  statusPrep_c4 : Constant  Value=15
  out_preppedBatch : Outport  PortName=preppedBatch  Element=batchId
  preppedBatch_el2 : Outport  PortName=preppedBatch  Element=recipeId
  preppedBatch_el3 : Outport  PortName=preppedBatch  Element=mass_kg
  preppedBatch_el4 : Outport  PortName=preppedBatch  Element=flow_bps
  out_statusPrep : Outport  Port=2  PortName=statusPrep  Element=unitId
  statusPrep_el2 : Outport  Port=2  PortName=statusPrep  Element=opState
  statusPrep_el3 : Outport  Port=2  PortName=statusPrep  Element=faultCode
  statusPrep_el4 : Outport  Port=2  PortName=statusPrep  Element=power_kW
  statusPrep_el5 : Outport  Port=2  PortName=statusPrep  Element=health
  wires:
  preppedBatch_c1/1 -> out_preppedBatch/1
  statusPrep_c1/1 -> out_statusPrep/1
  statusPrep_c3/1 -> statusPrep_el3/1
  RecipeClock/1 -> BlockIndex/1
  Gate_Fault_T_Cell2/1 -> En_Gate_Fault_T_Cell2/2, statusPrep_el5/1
  in_stagedIngredients/1 -> ThirdShare/1
  statusPrep_c2/1 -> statusPrep_el2/1
  Prep/1 -> preppedBatch_el4/1, ToKgPerHr/1
  in_directive/1 -> En_Gate_Fault_T_Cell2/1
  En_Gate_Fault_T_Cell2/1 -> Prep/2
  statusPrep_c4/1 -> statusPrep_el4/1
  ThirdShare/1 -> Prep/1
  BlockIndex/1 -> BlockFloor/1
  Prep/2 -> Trm46/1
  BlockFloor/1 -> RecipeMod/1
  RecipeCount/1 -> RecipeMod/2
  ToKgPerHr/1 -> preppedBatch_el3/1
  RecipeMod/1 -> RecipeBias/1
  RecipeBias/1 -> preppedBatch_el2/1

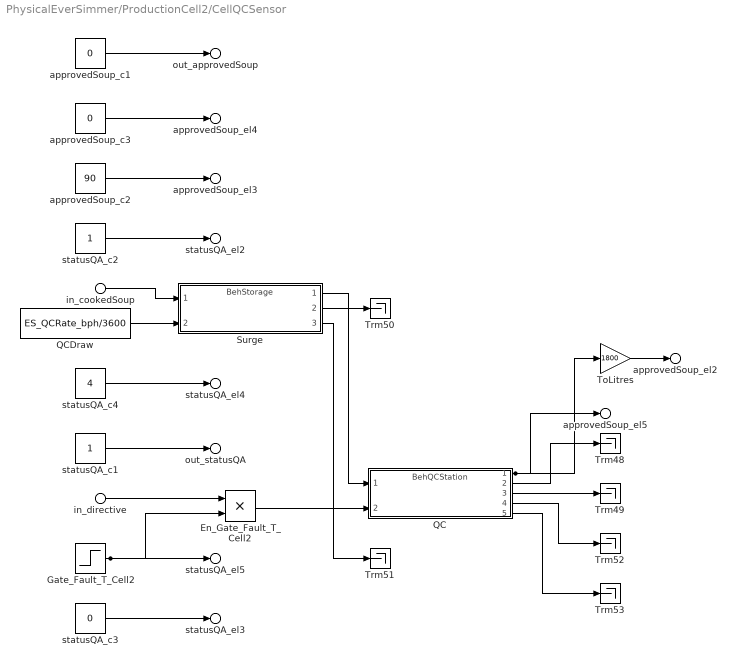
== system PhysicalEverSimmer/ProductionCell2/CellQCSensor ==
  in_cookedSoup : Inport  PortName=cookedSoup  Element=flow_bps
  in_directive : Inport  Port=2  PortName=directive  Element=setpoint
  En_Gate_Fault_T_Cell2 : Product
  Gate_Fault_T_Cell2 : Step  Time=Fault_T_Cell2  InitialValue=1  FinalValue=0  SampleTime=0
  QC : ModelReference  ModelNameDialog=BehQCStation  UsingDefaultArgumentValue=0,0,0,0,0,0  SimulationMode=Normal  ModelReferenceVersion=1.6
  QCDraw : Constant  Value=ES_QCRate_bph/3600
  Surge : ModelReference  ModelNameDialog=BehStorage  UsingDefaultArgumentValue=0,0  SimulationMode=Normal  ModelReferenceVersion=1.4
  ToLitres : Gain  Gain=1800
  Trm{48..53} (6 alike) : Terminator
  approvedSoup_c1 : Constant  Value=0
  approvedSoup_c2 : Constant  Value=90
  approvedSoup_c3 : Constant  Value=0
  statusQA_c1 : Constant
  statusQA_c2 : Constant
  statusQA_c3 : Constant  Value=0
  statusQA_c4 : Constant  Value=4
  out_approvedSoup : Outport  PortName=approvedSoup  Element=batchId
  approvedSoup_el2 : Outport  PortName=approvedSoup  Element=volume_L
  approvedSoup_el3 : Outport  PortName=approvedSoup  Element=temp_C
  approvedSoup_el4 : Outport  PortName=approvedSoup  Element=contamination_ppm
  approvedSoup_el5 : Outport  PortName=approvedSoup  Element=flow_bps
  out_statusQA : Outport  Port=2  PortName=statusQA  Element=unitId
  statusQA_el2 : Outport  Port=2  PortName=statusQA  Element=opState
  statusQA_el3 : Outport  Port=2  PortName=statusQA  Element=faultCode
  statusQA_el4 : Outport  Port=2  PortName=statusQA  Element=power_kW
  statusQA_el5 : Outport  Port=2  PortName=statusQA  Element=health
  wires:
  in_cookedSoup/1 -> Surge/1
  approvedSoup_c1/1 -> out_approvedSoup/1
  approvedSoup_c3/1 -> approvedSoup_el4/1
  QCDraw/1 -> Surge/2
  ToLitres/1 -> approvedSoup_el2/1
  approvedSoup_c2/1 -> approvedSoup_el3/1
  statusQA_c2/1 -> statusQA_el2/1
  statusQA_c4/1 -> statusQA_el4/1
  QC/5 -> Trm53/1
  statusQA_c1/1 -> out_statusQA/1
  En_Gate_Fault_T_Cell2/1 -> QC/2
  in_directive/1 -> En_Gate_Fault_T_Cell2/1
  Gate_Fault_T_Cell2/1 -> statusQA_el5/1, En_Gate_Fault_T_Cell2/2
  statusQA_c3/1 -> statusQA_el3/1
  Surge/1 -> QC/1
  Surge/2 -> Trm50/1
  Surge/3 -> Trm51/1
  QC/1 -> approvedSoup_el5/1, ToLitres/1
  QC/2 -> Trm48/1
  QC/3 -> Trm49/1
  QC/4 -> Trm52/1

== system PhysicalEverSimmer/ProductionCell3/CellController ==
  in_directive : Inport  PortName=directive
  statusPrepPwr : Inport  Port=2  PortName=statusPrep  Element=power_kW
  in_statusPrep : Inport  Port=2  PortName=statusPrep  Element=health
  statusCookPwr : Inport  Port=3  PortName=statusCook  Element=power_kW
  in_statusCook : Inport  Port=3  PortName=statusCook  Element=health
  statusQAPwr : Inport  Port=4  PortName=statusQA  Element=power_kW
  in_statusQA : Inport  Port=4  PortName=statusQA  Element=health
  statusPackPwr : Inport  Port=5  PortName=statusPack  Element=power_kW
  in_statusPack : Inport  Port=5  PortName=statusPack  Element=health
  HealthMin : MinMax  Inputs=4
  OwnPower : Constant  Value=2
  PowerSum : Sum  Inputs=+++++
  cellDirective_c1 : Constant  Value=0
  cellDirective_c2 : Constant  Value=0
  cellDirective_c3 : Constant
  statusCell_c1 : Constant  Value=3
  statusCell_c2 : Constant
  statusCell_c3 : Constant  Value=0
  out_cellDirective : Outport  PortName=cellDirective  Element=cmdType
  cellDirective_el2 : Outport  PortName=cellDirective  Element=targetId
  cellDirective_el3 : Outport  PortName=cellDirective  Element=setpoint
  out_statusCell : Outport  Port=2  PortName=statusCell  Element=unitId
  statusCell_el2 : Outport  Port=2  PortName=statusCell  Element=opState
  statusCell_el3 : Outport  Port=2  PortName=statusCell  Element=faultCode
  statusCell_el4 : Outport  Port=2  PortName=statusCell  Element=power_kW
  statusCell_el5 : Outport  Port=2  PortName=statusCell  Element=health
  wires:
  cellDirective_c1/1 -> out_cellDirective/1
  cellDirective_c2/1 -> cellDirective_el2/1
  statusCell_c2/1 -> statusCell_el2/1
  statusQAPwr/1 -> PowerSum/3
  statusPrepPwr/1 -> PowerSum/1
  cellDirective_c3/1 -> cellDirective_el3/1
  statusCell_c3/1 -> statusCell_el3/1
  statusCookPwr/1 -> PowerSum/2
  statusPackPwr/1 -> PowerSum/4
  OwnPower/1 -> PowerSum/5
  in_statusPrep/1 -> HealthMin/1
  in_statusCook/1 -> HealthMin/2
  in_statusQA/1 -> HealthMin/3
  in_statusPack/1 -> HealthMin/4
  statusCell_c1/1 -> out_statusCell/1
  PowerSum/1 -> statusCell_el4/1
  HealthMin/1 -> statusCell_el5/1

== system PhysicalEverSimmer/ProductionCell3/CellCookVat ==
  in_preppedBatch : Inport  PortName=preppedBatch  Element=flow_bps
  in_directive : Inport  Port=2  PortName=directive  Element=setpoint
  En_Gate_Fault_T_Cell3 : Product
  Gate_Fault_T_Cell3 : Step  Time=Fault_T_Cell3  InitialValue=1  FinalValue=0  SampleTime=0
  StateDbl : DataTypeConversion  OutDataTypeStr=double  SaturateOnIntegerOverflow=off  RndMeth=Floor
  ToLitres : Gain  Gain=1800
  Trm57 : Terminator
  Vat : ModelReference  ModelNameDialog=BehCookVat  UsingDefaultArgumentValue=0,0,0,0,0,0,0,0  SimulationMode=Normal  ModelReferenceVersion=1.15
  cookedSoup_c1 : Constant  Value=0
  cookedSoup_c2 : Constant  Value=0
  statusCook_c1 : Constant  Value=3
  statusCook_c2 : Constant  Value=0
  out_cookedSoup : Outport  PortName=cookedSoup  Element=batchId
  cookedSoup_el2 : Outport  PortName=cookedSoup  Element=volume_L
  cookedSoup_el3 : Outport  PortName=cookedSoup  Element=temp_C
  cookedSoup_el4 : Outport  PortName=cookedSoup  Element=contamination_ppm
  cookedSoup_el5 : Outport  PortName=cookedSoup  Element=flow_bps
  out_statusCook : Outport  Port=2  PortName=statusCook  Element=unitId
  statusCook_el2 : Outport  Port=2  PortName=statusCook  Element=opState
  statusCook_el3 : Outport  Port=2  PortName=statusCook  Element=faultCode
  statusCook_el4 : Outport  Port=2  PortName=statusCook  Element=power_kW
  statusCook_el5 : Outport  Port=2  PortName=statusCook  Element=health
  wires:
  statusCook_c2/1 -> statusCook_el3/1
  cookedSoup_c2/1 -> cookedSoup_el4/1
  Vat/3 -> cookedSoup_el3/1
  En_Gate_Fault_T_Cell3/1 -> Vat/2
  in_preppedBatch/1 -> Vat/1
  ToLitres/1 -> cookedSoup_el2/1
  statusCook_c1/1 -> out_statusCook/1
  cookedSoup_c1/1 -> out_cookedSoup/1
  in_directive/1 -> En_Gate_Fault_T_Cell3/1
  Gate_Fault_T_Cell3/1 -> En_Gate_Fault_T_Cell3/2, statusCook_el5/1
  Vat/1 -> cookedSoup_el5/1, ToLitres/1  "soupFlow_Cell3"
  Vat/2 -> statusCook_el4/1
  Vat/4 -> StateDbl/1
  Vat/5 -> Trm57/1
  StateDbl/1 -> statusCook_el2/1

== system PhysicalEverSimmer/ProductionCell3/CellPackager ==
  in_approvedSoup : Inport  PortName=approvedSoup  Element=flow_bps
  in_directive : Inport  Port=2  PortName=directive  Element=setpoint
  En_Gate_Fault_T_Cell3 : Product
  Gate_Fault_T_Cell3 : Step  Time=Fault_T_Cell3  InitialValue=1  FinalValue=0  SampleTime=0
  Pack : ModelReference  ModelNameDialog=BehPackager  UsingDefaultArgumentValue=0,0  SimulationMode=Normal  ModelReferenceVersion=1.5
  PackDraw : Constant  Value=ES_PackRate_bph/3600
  Surge : ModelReference  ModelNameDialog=BehStorage  UsingDefaultArgumentValue=0,0  SimulationMode=Normal  ModelReferenceVersion=1.4
  Trm64 : Terminator
  Trm65 : Terminator
  sealedContainers_c1 : Constant  Value=0
  sealedContainers_c2 : Constant  Value=0
  sealedContainers_c3 : Constant  Value=365
  statusPack_c1 : Constant
  statusPack_c2 : Constant
  statusPack_c3 : Constant  Value=0
  statusPack_c4 : Constant  Value=12
  out_sealedContainers : Outport  PortName=sealedContainers  Element=batchId
  sealedContainers_el2 : Outport  PortName=sealedContainers  Element=count
  sealedContainers_el3 : Outport  PortName=sealedContainers  Element=sealRating_days
  sealedContainers_el4 : Outport  PortName=sealedContainers  Element=flow_bps
  out_statusPack : Outport  Port=2  PortName=statusPack  Element=unitId
  statusPack_el2 : Outport  Port=2  PortName=statusPack  Element=opState
  statusPack_el3 : Outport  Port=2  PortName=statusPack  Element=faultCode
  statusPack_el4 : Outport  Port=2  PortName=statusPack  Element=power_kW
  statusPack_el5 : Outport  Port=2  PortName=statusPack  Element=health
  wires:
  statusPack_c2/1 -> statusPack_el2/1
  En_Gate_Fault_T_Cell3/1 -> Pack/2
  in_directive/1 -> En_Gate_Fault_T_Cell3/1
  sealedContainers_c3/1 -> sealedContainers_el3/1
  sealedContainers_c1/1 -> out_sealedContainers/1
  statusPack_c4/1 -> statusPack_el4/1
  in_approvedSoup/1 -> Surge/1
  statusPack_c1/1 -> out_statusPack/1
  Gate_Fault_T_Cell3/1 -> En_Gate_Fault_T_Cell3/2, statusPack_el5/1
  statusPack_c3/1 -> statusPack_el3/1
  PackDraw/1 -> Surge/2
  sealedContainers_c2/1 -> sealedContainers_el2/1
  Surge/1 -> Pack/1
  Surge/2 -> Trm64/1
  Surge/3 -> Trm65/1
  Pack/1 -> sealedContainers_el4/1

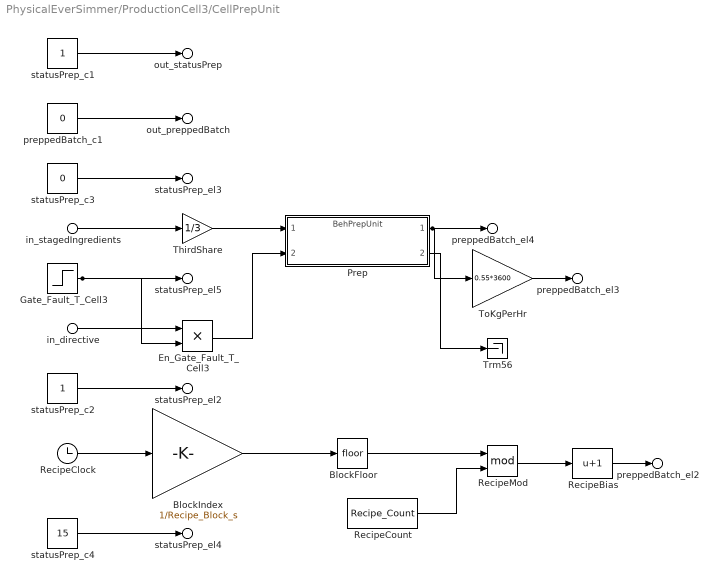
== system PhysicalEverSimmer/ProductionCell3/CellPrepUnit ==
  in_stagedIngredients : Inport  PortName=stagedIngredients  Element=flow_bps
  in_directive : Inport  Port=2  PortName=directive  Element=setpoint
  BlockFloor : Rounding
  BlockIndex : Gain  Gain=1/Recipe_Block_s
  En_Gate_Fault_T_Cell3 : Product
  Gate_Fault_T_Cell3 : Step  Time=Fault_T_Cell3  InitialValue=1  FinalValue=0  SampleTime=0
  Prep : ModelReference  ModelNameDialog=BehPrepUnit  UsingDefaultArgumentValue=0,0  SimulationMode=Normal  ModelReferenceVersion=1.5
  RecipeBias : Bias  Bias=1  SaturateOnIntegerOverflow=off
  RecipeClock : Clock
  RecipeCount : Constant  Value=Recipe_Count
  RecipeMod : Math  Operator=mod
  ThirdShare : Gain  Gain=1/3
  ToKgPerHr : Gain  Gain=0.55*3600
  Trm56 : Terminator
  preppedBatch_c1 : Constant  Value=0
  statusPrep_c1 : Constant
  statusPrep_c2 : Constant
  statusPrep_c3 : Constant  Value=0
  statusPrep_c4 : Constant  Value=15
  out_preppedBatch : Outport  PortName=preppedBatch  Element=batchId
  preppedBatch_el2 : Outport  PortName=preppedBatch  Element=recipeId
  preppedBatch_el3 : Outport  PortName=preppedBatch  Element=mass_kg
  preppedBatch_el4 : Outport  PortName=preppedBatch  Element=flow_bps
  out_statusPrep : Outport  Port=2  PortName=statusPrep  Element=unitId
  statusPrep_el2 : Outport  Port=2  PortName=statusPrep  Element=opState
  statusPrep_el3 : Outport  Port=2  PortName=statusPrep  Element=faultCode
  statusPrep_el4 : Outport  Port=2  PortName=statusPrep  Element=power_kW
  statusPrep_el5 : Outport  Port=2  PortName=statusPrep  Element=health
  wires:
  in_directive/1 -> En_Gate_Fault_T_Cell3/1
  Prep/1 -> preppedBatch_el4/1, ToKgPerHr/1
  statusPrep_c1/1 -> out_statusPrep/1
  statusPrep_c2/1 -> statusPrep_el2/1
  preppedBatch_c1/1 -> out_preppedBatch/1
  RecipeClock/1 -> BlockIndex/1
  Gate_Fault_T_Cell3/1 -> En_Gate_Fault_T_Cell3/2, statusPrep_el5/1
  in_stagedIngredients/1 -> ThirdShare/1
  statusPrep_c3/1 -> statusPrep_el3/1
  statusPrep_c4/1 -> statusPrep_el4/1
  ThirdShare/1 -> Prep/1
  En_Gate_Fault_T_Cell3/1 -> Prep/2
  BlockIndex/1 -> BlockFloor/1
  Prep/2 -> Trm56/1
  BlockFloor/1 -> RecipeMod/1
  RecipeCount/1 -> RecipeMod/2
  ToKgPerHr/1 -> preppedBatch_el3/1
  RecipeMod/1 -> RecipeBias/1
  RecipeBias/1 -> preppedBatch_el2/1

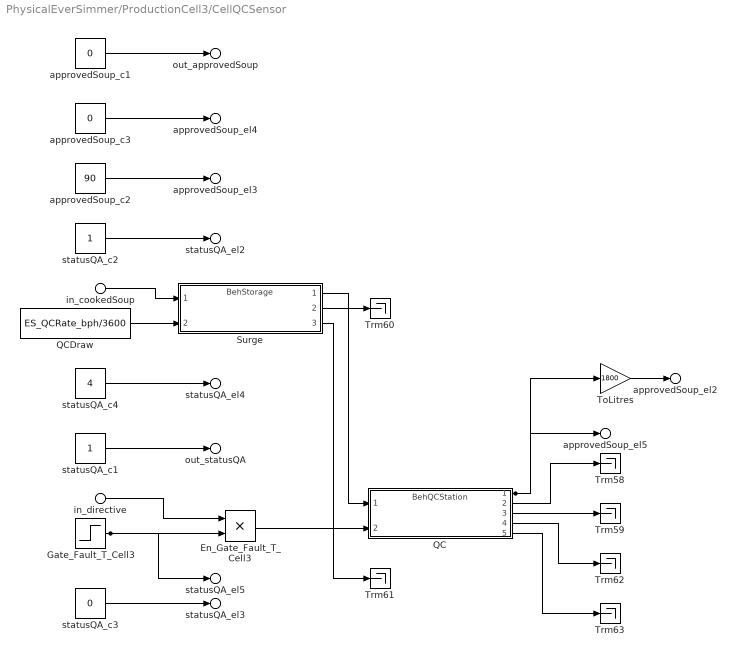
== system PhysicalEverSimmer/ProductionCell3/CellQCSensor ==
  in_cookedSoup : Inport  PortName=cookedSoup  Element=flow_bps
  in_directive : Inport  Port=2  PortName=directive  Element=setpoint
  En_Gate_Fault_T_Cell3 : Product
  Gate_Fault_T_Cell3 : Step  Time=Fault_T_Cell3  InitialValue=1  FinalValue=0  SampleTime=0
  QC : ModelReference  ModelNameDialog=BehQCStation  UsingDefaultArgumentValue=0,0,0,0,0,0  SimulationMode=Normal  ModelReferenceVersion=1.6
  QCDraw : Constant  Value=ES_QCRate_bph/3600
  Surge : ModelReference  ModelNameDialog=BehStorage  UsingDefaultArgumentValue=0,0  SimulationMode=Normal  ModelReferenceVersion=1.4
  ToLitres : Gain  Gain=1800
  Trm{58..63} (6 alike) : Terminator
  approvedSoup_c1 : Constant  Value=0
  approvedSoup_c2 : Constant  Value=90
  approvedSoup_c3 : Constant  Value=0
  statusQA_c1 : Constant
  statusQA_c2 : Constant
  statusQA_c3 : Constant  Value=0
  statusQA_c4 : Constant  Value=4
  out_approvedSoup : Outport  PortName=approvedSoup  Element=batchId
  approvedSoup_el2 : Outport  PortName=approvedSoup  Element=volume_L
  approvedSoup_el3 : Outport  PortName=approvedSoup  Element=temp_C
  approvedSoup_el4 : Outport  PortName=approvedSoup  Element=contamination_ppm
  approvedSoup_el5 : Outport  PortName=approvedSoup  Element=flow_bps
  out_statusQA : Outport  Port=2  PortName=statusQA  Element=unitId
  statusQA_el2 : Outport  Port=2  PortName=statusQA  Element=opState
  statusQA_el3 : Outport  Port=2  PortName=statusQA  Element=faultCode
  statusQA_el4 : Outport  Port=2  PortName=statusQA  Element=power_kW
  statusQA_el5 : Outport  Port=2  PortName=statusQA  Element=health
  wires:
  in_cookedSoup/1 -> Surge/1
  approvedSoup_c1/1 -> out_approvedSoup/1
  approvedSoup_c3/1 -> approvedSoup_el4/1
  QCDraw/1 -> Surge/2
  approvedSoup_c2/1 -> approvedSoup_el3/1
  statusQA_c2/1 -> statusQA_el2/1
  statusQA_c4/1 -> statusQA_el4/1
  statusQA_c1/1 -> out_statusQA/1
  in_directive/1 -> En_Gate_Fault_T_Cell3/1
  Gate_Fault_T_Cell3/1 -> En_Gate_Fault_T_Cell3/2, statusQA_el5/1
  statusQA_c3/1 -> statusQA_el3/1
  Surge/1 -> QC/1
  Surge/2 -> Trm60/1
  Surge/3 -> Trm61/1
  En_Gate_Fault_T_Cell3/1 -> QC/2
  QC/1 -> approvedSoup_el5/1, ToLitres/1
  QC/2 -> Trm58/1
  QC/3 -> Trm59/1
  QC/4 -> Trm62/1
  QC/5 -> Trm63/1
  ToLitres/1 -> approvedSoup_el2/1
